simulink model "OfficeChairIntegratorsT4MarcelM"  (R2023a)
settings: Solver=VariableStepAuto  StartTime=0.0  StopTime=10.0  RelTol=1e-3
undefined symbols (not defined in the file): b, g, k, m, M
settings Model: Creator=marcelmartens  LastModifiedBy=marcelmartens

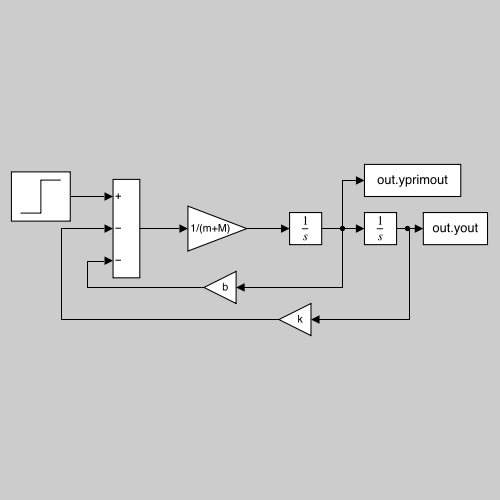
[thumbnail: Simulink's stored preview of the top-level diagram]
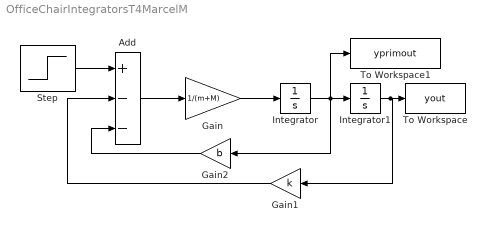
== system OfficeChairIntegratorsT4MarcelM ==
  Add : Sum  Inputs=+--
  Gain : Gain  Gain=1/(m+M)
  Gain1 : Gain  Gain=k
  Gain2 : Gain  Gain=b
  Integrator : Integrator
  Integrator1 : Integrator
  Step : Step  Time=0  After=M*g  SampleTime=0
  To Workspace : ToWorkspace  VariableName=yout  SaveFormat=Timeseries  SampleTime=-1
  To Workspace1 : ToWorkspace  VariableName=yprimout  SaveFormat=Timeseries  SampleTime=-1
  wires:
  Integrator1/1 -> To Workspace/1, Gain1/1
  Integrator/1 -> To Workspace1/1, Gain2/1, Integrator1/1
  Step/1 -> Add/1
  Gain1/1 -> Add/2
  Gain/1 -> Integrator/1
  Gain2/1 -> Add/3
  Add/1 -> Gain/1
